simulink library "acc"  (R2021b)
settings: Solver=VariableStepAuto  StartTime=0.0  StopTime=10.0  RelTol=1e-3
undefined symbols (not defined in the file or in its folder): AACC_EHPSSpdCtrlMode_X_enum, AACC_EHPSSpdCtrlMode_Y_rad, ENUM__SASCALED_CALED, ENUM_BRAKEPEDAL_RELEASED, ENUM_CACENABLESTS_RUN, ENUM_DCDCENABLESTS_RUN, ENUM_EHPSCTRLMODE_FULLPWR, ENUM_EHPSCTRLMODE_NORMAL, ENUM_EHPSCTRLMODE_STEP1, ENUM_EHPSCTRLMODE_ZERO, ENUM_EHPSENABLESTS_INITIAL, ENUM_EHPSENABLESTS_READY, ENUM_EHPSENABLESTS_RUN, ENUM_PMMMODE_DRIVE, ENUM_PMMMODE_POWERUP, ENUM_TARGETGEAR_NEUTRAL, FALSE, KACC_AirPressInvalid_kpa, KACC_CACEnableFailTime_s, KACC_CACOverrunRcvTime_s, KACC_CACOverrunTime_min, KACC_CACOverTempDelayTime_s, KACC_CACOverTempRcv_s, KACC_CACPresLow_kPa, KACC_CACPressureSWRev_flg, KACC_CACPresWarn_kPa, KACC_CACPresWarn_ovrdflg_flg, KACC_CACPresWarn_ovrdval_flg, KACC_CACStopTime_s, KACC_CACTemp_C, KACC_CACTempRev_C, KACC_CACTempStop_C, KACC_CACTempWarn_C, KACC_CACValid_flg, KACC_CP2VAutoTracH_enum, KACC_CP2VDamStiffReqFA_pct, KACC_CP2VDamStiffReqLA_pct, KACC_CP2VDamStiffReqRA_pct, KACC_CP2VKneeCtrlMReq_enum, KACC_CP2VKneeReqFA_enum, KACC_CP2VKneeReqRA_enum, KACC_CP2VKneeReqRSide_enum, KACC_CP2VLA1PosCmd_enum, KACC_CP2VLA2PosCmd_enum, KACC_CP2VLvCtrlModeReq_enum, KACC_CP2VNLvReqFA_enum, KACC_CP2VNLvReqRA_enum, KACC_DCDCErrLvHoldtime_s, KACC_DTCACCReset_flg, KACC_DTCCACOverrun_cnt, KACC_EACErrLvHoldtime_s, KACC_ECASKneeSideSW_flg, KACC_EcasSw1Down_flg, KACC_EcasSw1Up_flg, KACC_EcasSw2M2_flg, KACC_EcasSw2Stop_flg, KACC_EcasSw3Knee_flg, KACC_EcasSw3M1_flg, KACC_EcasSwDebounceTime_s, KACC_ECASSwitch_flg ... (+30)
libraries: hcu_lib x20, simulink x3
(part 3 of 3)

== system acc/ACC/OutpConvert/EHPS Enable TimeOut Judgment ==
  BSCP_In_outputs : Inport
  BMain_outputs : Inport  Port=2
  Bus Selector : BusSelector  OutputSignals=VPMM_EHPSIniFinish_flg,VINP_EHPSEnSta_enum,task_time_s
  Bus Selector1 : BusSelector  OutputSignals=VACC_InitEHPSEnDem_flg
  Constant19 : Constant  Value=ENUM_EHPSENABLESTS_INITIAL
  Constant20 : Constant  Value=KACC_EHPSDisableFailTime_s
  Constant21 : Constant  Value=ENUM_EHPSENABLESTS_READY
  DelayEnable1 : Subsystem  mask(DelayEnable){}
      mask help: Delay enable funcion.
  Logical Operator1 : Logic  Inputs=3  AllPortsSameDT=off  OutDataTypeStr=boolean
  Logical Operator3 : Logic  Operator=OR  AllPortsSameDT=off  OutDataTypeStr=boolean
  NOT1 : Logic  Operator=NOT  AllPortsSameDT=off  OutDataTypeStr=boolean
  Relational Operator7 : RelationalOperator  Operator=~=  OutDataTypeStr=boolean  RndMeth=Simplest
  Relational Operator8 : RelationalOperator  Operator=~=  OutDataTypeStr=boolean  RndMeth=Simplest
  Unit Delay3 : UnitDelay  InitialCondition=boolean(0)  SampleTime=-1  HasFrameUpgradeWarning=on
      settings: AttributesFormatString=%<InitialCondition>
  VACC_EHPSDisEnTimeout_flg : Outport
  wires:
  [task_time_s] -> DelayEnable1/3(Ts)
  [VINP_EHPSEnSta_enum] -> Relational Operator8/1
  DelayEnable1/1(set) -> Unit Delay3/1
  Relational Operator7/1 -> Logical Operator3/1
  Constant20/1 -> DelayEnable1/2(T_delay)
  Logical Operator3/1 -> Logical Operator1/3
  Constant21/1 -> Relational Operator8/2
  [VINP_EHPSEnSta_enum] -> Relational Operator7/1
  NOT1/1 -> Logical Operator1/2
  Constant19/1 -> Relational Operator7/2
  [VACC_InitEHPSEnDem_flg] -> NOT1/1
  [VPMM_EHPSIniFinish_flg] -> Logical Operator1/1
  Relational Operator8/1 -> Logical Operator3/2
  Logical Operator1/1 -> DelayEnable1/1(trigger)
  Bus Selector/1 -> [VPMM_EHPSIniFinish_flg]  "<VPMM_EHPSIniFinish_flg>"
  Bus Selector/2 -> [VINP_EHPSEnSta_enum]  "<VINP_EHPSEnSta_enum>"
  BSCP_In_outputs/1 -> Bus Selector/1
  BMain_outputs/1 -> Bus Selector1/1
  Bus Selector1/1 -> [VACC_InitEHPSEnDem_flg]  "<VACC_InitEHPSEnDem_flg>"
  Bus Selector/3 -> [task_time_s]  "<task_time_s>"
  Unit Delay3/1 -> [VACC_EHPSDisEnTimeout_flg]  "VACC_EHPSDisEnTimeout_flg"
  [VACC_EHPSDisEnTimeout_flg] -> VACC_EHPSDisEnTimeout_flg/1

== system acc/ACC/OutpConvert/PCU Demand SCP ==
  BMain_outputs : Inport
  Bus Selector1 : BusSelector  OutputSignals=VACC_EHPSEnableDem_flg,VACC_CACEnableDem_flg,VACC_DCDCEnableDem_flg
  Constant10 : Constant  Value=hex2dec('AA')  OutDataTypeStr=uint8
  Constant11 : Constant  Value=ZERO_FLOAT
  Constant12 : Constant  Value=ZERO_FLOAT
  Constant6 : Constant  Value=hex2dec('55')  OutDataTypeStr=uint8
  Constant7 : Constant  Value=hex2dec('AA')  OutDataTypeStr=uint8
  Constant8 : Constant  Value=hex2dec('55')  OutDataTypeStr=uint8
  Constant9 : Constant  Value=hex2dec('AA')  OutDataTypeStr=uint8
  Constant90 : Constant  Value=hex2dec('55')  OutDataTypeStr=uint8
  Data Type Conversion63 : DataTypeConversion  OutDataTypeStr=single
  Data Type Conversion64 : DataTypeConversion  OutDataTypeStr=single
  Switch : Switch  Criteria=u2 > Threshold
  Switch1 : Switch  Criteria=u2 > Threshold
  Switch2 : Switch  Criteria=u2 > Threshold
  Terminator : Terminator
  VACC_EHPSEnDemand_enum : Outport
  VACC_EACEnDemand_enum : Outport  Port=2
  VACC_DCDCEnDemamd_enum : Outport  Port=3
  VACC_EACSpdDemand_rpm : Outport  Port=4
  wires:
  Constant10/1 -> Switch2/3
  Constant9/1 -> Switch/3
  Constant11/1 -> Data Type Conversion64/1
  Constant6/1 -> Switch1/1
  Constant7/1 -> Switch1/3
  Constant12/1 -> Data Type Conversion63/1
  Data Type Conversion64/1 -> Terminator/1
  Constant90/1 -> Switch2/1
  Constant8/1 -> Switch/1
  BMain_outputs/1 -> Bus Selector1/1
  Bus Selector1/1 -> [VACC_EHPSEnableDem_flg]  "<VACC_EHPSEnableDem_flg>"
  Bus Selector1/2 -> [VACC_CACEnableDem_flg]  "<VACC_CACEnableDem_flg>"
  Bus Selector1/3 -> [VACC_DCDCEnableDem_flg]  "<VACC_DCDCEnableDem_flg>"
  [VACC_EHPSEnableDem_flg] -> Switch/2
  [VACC_DCDCEnableDem_flg] -> Switch2/2
  [VACC_CACEnableDem_flg] -> Switch1/2
  Switch/1 -> [VACC_EHPSEnDemand_enum]  "VACC_EHPSEnDemand_enum"
  Switch1/1 -> [VACC_EACEnDemand_enum]  "VACC_EACEnDemand_enum"
  Switch2/1 -> [VACC_DCDCEnDemamd_enum]  "VACC_DCDCEnDemamd_enum"
  Data Type Conversion63/1 -> [VACC_EACSpdDemand_rpm]  "VACC_EACSpdDemand_rpm"
  [VACC_EHPSEnDemand_enum] -> VACC_EHPSEnDemand_enum/1
  [VACC_EACEnDemand_enum] -> VACC_EACEnDemand_enum/1
  [VACC_DCDCEnDemamd_enum] -> VACC_DCDCEnDemamd_enum/1
  [VACC_EACSpdDemand_rpm] -> VACC_EACSpdDemand_rpm/1

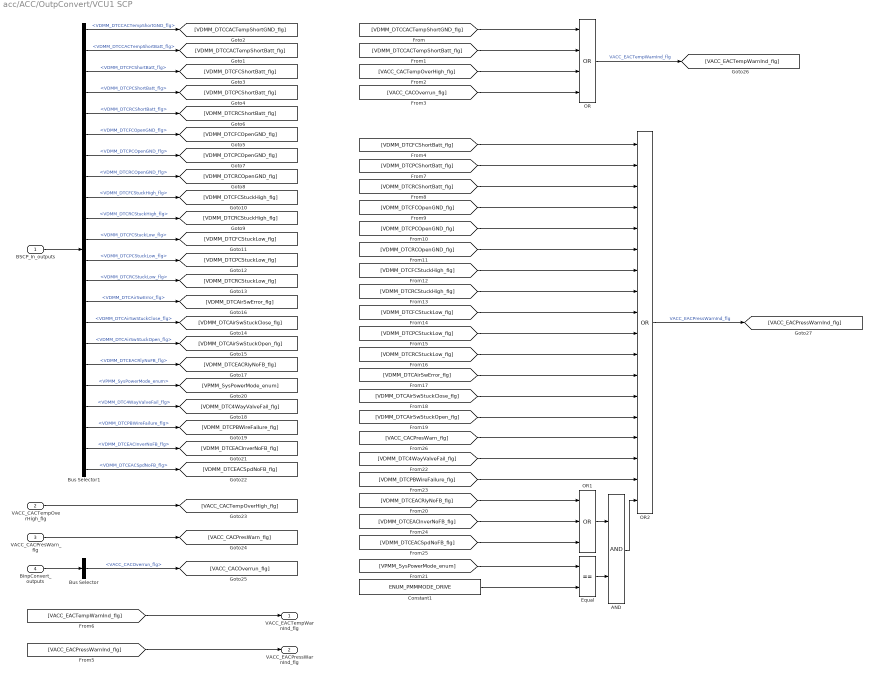
== system acc/ACC/OutpConvert/VCU1 SCP ==
  BSCP_In_outputs : Inport
  VACC_CACTempOverHigh_flg : Inport  Port=2
  VACC_CACPresWarn_flg : Inport  Port=3
  BInpConvert_outputs : Inport  Port=4
  AND : Logic  AllPortsSameDT=off  OutDataTypeStr=boolean
  Bus Selector : BusSelector  OutputSignals=VACC_CACOverrun_flg
  Bus Selector1 : BusSelector  OutputSignals=VDMM_DTCCACTempShortGND_flg,VDMM_DTCCACTempShortBatt_flg,VDMM_DTCFCShortBatt_flg,VDMM_DTCPCShortBatt_flg,VDMM_DTCRCShortBatt_flg,VDMM_DTCFCOpenGND_flg,VDMM_DTCPCOpenGND_flg,VDMM_DTCRCOpenGND_flg,VDMM_DTCFCStuckHigh_flg,VDMM_DTCRCStuckHigh_flg,VDMM_DTCFCStuckLow_flg,VDMM_DTCPCStuckLow_flg,VDMM_DTCRCStuckLow_flg,VDMM_DTCAirSwError_flg,VDMM_DTCAirSwStuckClose_flg,VDMM_DTCAirSwStuckOpen_flg,VDMM_DTCEACRlyNoFB_flg,VPMM_SysPowerMode_enum,VDMM_DTC4WayValveFail_flg,VDMM_DTCPBWireFailure_flg,VDMM_DTCEACInverNoFB_flg,VDMM_DTCEACSpdNoFB_flg
  Constant1 : Constant  Value=ENUM_PMMMODE_DRIVE
  Equal : RelationalOperator  Operator===  OutDataTypeStr=boolean  RndMeth=Simplest
  OR : Logic  Operator=OR  Inputs=4  AllPortsSameDT=off  OutDataTypeStr=boolean
  OR1 : Logic  Operator=OR  Inputs=3  AllPortsSameDT=off  OutDataTypeStr=boolean
  OR2 : Logic  Operator=OR  Inputs=18  AllPortsSameDT=off  OutDataTypeStr=boolean
  VACC_EACTempWarnInd_flg : Outport
  VACC_EACPressWarnInd_flg : Outport  Port=2
  wires:
  [VACC_EACPressWarnInd_flg] -> VACC_EACPressWarnInd_flg/1
  [VACC_EACTempWarnInd_flg] -> VACC_EACTempWarnInd_flg/1
  BSCP_In_outputs/1 -> Bus Selector1/1
  Bus Selector1/4 -> [VDMM_DTCPCShortBatt_flg]  "<VDMM_DTCPCShortBatt_flg>"
  Bus Selector1/3 -> [VDMM_DTCFCShortBatt_flg]  "<VDMM_DTCFCShortBatt_flg>"
  Bus Selector1/2 -> [VDMM_DTCCACTempShortBatt_flg]  "<VDMM_DTCCACTempShortBatt_flg>"
  Bus Selector1/1 -> [VDMM_DTCCACTempShortGND_flg]  "<VDMM_DTCCACTempShortGND_flg>"
  Bus Selector1/5 -> [VDMM_DTCRCShortBatt_flg]  "<VDMM_DTCRCShortBatt_flg>"
  Bus Selector1/6 -> [VDMM_DTCFCOpenGND_flg]  "<VDMM_DTCFCOpenGND_flg>"
  Bus Selector1/7 -> [VDMM_DTCPCOpenGND_flg]  "<VDMM_DTCPCOpenGND_flg>"
  Bus Selector1/8 -> [VDMM_DTCRCOpenGND_flg]  "<VDMM_DTCRCOpenGND_flg>"
  Bus Selector1/9 -> [VDMM_DTCFCStuckHigh_flg]  "<VDMM_DTCFCStuckHigh_flg>"
  Bus Selector1/10 -> [VDMM_DTCRCStuckHigh_flg]  "<VDMM_DTCRCStuckHigh_flg>"
  Bus Selector1/11 -> [VDMM_DTCFCStuckLow_flg]  "<VDMM_DTCFCStuckLow_flg>"
  Bus Selector1/12 -> [VDMM_DTCPCStuckLow_flg]  "<VDMM_DTCPCStuckLow_flg>"
  Bus Selector1/13 -> [VDMM_DTCRCStuckLow_flg]  "<VDMM_DTCRCStuckLow_flg>"
  Bus Selector1/14 -> [VDMM_DTCAirSwError_flg]  "<VDMM_DTCAirSwError_flg>"
  Bus Selector1/15 -> [VDMM_DTCAirSwStuckClose_flg]  "<VDMM_DTCAirSwStuckClose_flg>"
  Bus Selector1/16 -> [VDMM_DTCAirSwStuckOpen_flg]  "<VDMM_DTCAirSwStuckOpen_flg>"
  Bus Selector1/17 -> [VDMM_DTCEACRlyNoFB_flg]  "<VDMM_DTCEACRlyNoFB_flg>"
  Bus Selector1/18 -> [VPMM_SysPowerMode_enum]  "<VPMM_SysPowerMode_enum>"
  Bus Selector1/19 -> [VDMM_DTC4WayValveFail_flg]  "<VDMM_DTC4WayValveFail_flg>"
  Bus Selector1/20 -> [VDMM_DTCPBWireFailure_flg]  "<VDMM_DTCPBWireFailure_flg>"
  Bus Selector1/21 -> [VDMM_DTCEACInverNoFB_flg]  "<VDMM_DTCEACInverNoFB_flg>"
  Bus Selector1/22 -> [VDMM_DTCEACSpdNoFB_flg]  "<VDMM_DTCEACSpdNoFB_flg>"
  BInpConvert_outputs/1 -> Bus Selector/1
  Bus Selector/1 -> [VACC_CACOverrun_flg]  "<VACC_CACOverrun_flg>"
  VACC_CACPresWarn_flg/1 -> [VACC_CACPresWarn_flg]
  VACC_CACTempOverHigh_flg/1 -> [VACC_CACTempOverHigh_flg]
  [VDMM_DTCCACTempShortGND_flg] -> OR/1
  [VDMM_DTCCACTempShortBatt_flg] -> OR/2
  [VACC_CACTempOverHigh_flg] -> OR/3
  [VACC_CACOverrun_flg] -> OR/4
  OR/1 -> [VACC_EACTempWarnInd_flg]  "VACC_EACTempWarnInd_flg"
  Constant1/1 -> Equal/2
  [VPMM_SysPowerMode_enum] -> Equal/1
  [VDMM_DTCEACRlyNoFB_flg] -> OR1/1
  [VDMM_DTCEACInverNoFB_flg] -> OR1/2
  [VDMM_DTCEACSpdNoFB_flg] -> OR1/3
  OR1/1 -> AND/1
  Equal/1 -> AND/2
  [VDMM_DTCFCShortBatt_flg] -> OR2/1
  [VDMM_DTCPCShortBatt_flg] -> OR2/2
  [VDMM_DTCRCShortBatt_flg] -> OR2/3
  [VDMM_DTCFCOpenGND_flg] -> OR2/4
  [VDMM_DTCPCOpenGND_flg] -> OR2/5
  [VDMM_DTCRCOpenGND_flg] -> OR2/6
  [VDMM_DTCFCStuckHigh_flg] -> OR2/7
  [VDMM_DTCRCStuckHigh_flg] -> OR2/8
  [VDMM_DTCFCStuckLow_flg] -> OR2/9
  [VDMM_DTCPCStuckLow_flg] -> OR2/10
  [VDMM_DTCRCStuckLow_flg] -> OR2/11
  [VDMM_DTCAirSwError_flg] -> OR2/12
  [VDMM_DTCAirSwStuckClose_flg] -> OR2/13
  [VDMM_DTCAirSwStuckOpen_flg] -> OR2/14
  [VACC_CACPresWarn_flg] -> OR2/15
  [VDMM_DTC4WayValveFail_flg] -> OR2/16
  [VDMM_DTCPBWireFailure_flg] -> OR2/17
  AND/1 -> OR2/18
  OR2/1 -> [VACC_EACPressWarnInd_flg]  "VACC_EACPressWarnInd_flg"

== system acc/ACC/OutpConvert/VCU5 SCP ==
  BSCP_In_outputs : Inport
  Bus Selector1 : BusSelector  OutputSignals=VINP_CACTemp_C,VINP_FDCCHASSISVCUEACPressSta_flg,VDMM_DTCCACTempShortGND_flg,VDMM_DTCCACTempShortBatt_flg
  Constant1 : Constant  Value=KACC_CACPressureSWRev_flg
  Constant21 : Constant  Value=KACC_VCUEACpumpTempInvalid_C
  NOT : Logic  Operator=NOT  AllPortsSameDT=off  OutDataTypeStr=boolean
  OR : Logic  Operator=OR  AllPortsSameDT=off  OutDataTypeStr=boolean
  Switch : Switch  Criteria=u2 ~= 0
      settings: AttributesFormatString=%<Criteria>
  Switch1 : Switch  Criteria=u2 ~= 0
      settings: AttributesFormatString=%<Criteria>
  VACC_VCUEACpumpTemp_C : Outport
  VACC_VCUEACPressureSW_flg : Outport  Port=2
  wires:
  BSCP_In_outputs/1 -> Bus Selector1/1
  Bus Selector1/1 -> [VINP_CACTemp_C]  "<VINP_CACTemp_C>"
  Bus Selector1/2 -> [VINP_FDCCHASSISVCUEACPressSta_flg]  "<VINP_FDCCHASSISVCUEACPressSta_flg>"
  Bus Selector1/3 -> [VDMM_DTCCACTempShortGND_flg]  "<VDMM_DTCCACTempShortGND_flg>"
  Bus Selector1/4 -> [VDMM_DTCCACTempShortBatt_flg]  "<VDMM_DTCCACTempShortBatt_flg>"
  OR/1 -> Switch/2
  [VDMM_DTCCACTempShortGND_flg] -> OR/1
  [VDMM_DTCCACTempShortBatt_flg] -> OR/2
  Constant21/1 -> Switch/1
  [VINP_CACTemp_C] -> Switch/3
  Switch/1 -> [VACC_VCUEACpumpTemp_C]  "VACC_VCUEACpumpTemp_C"
  Constant1/1 -> Switch1/2
  [VINP_FDCCHASSISVCUEACPressSta_flg] -> NOT/1
  NOT/1 -> Switch1/3
  [VINP_FDCCHASSISVCUEACPressSta_flg] -> Switch1/1
  Switch1/1 -> [VACC_VCUEACPressureSW_flg]  "VACC_VCUEACPressureSW_flg"
  [VACC_VCUEACpumpTemp_C] -> VACC_VCUEACpumpTemp_C/1
  [VACC_VCUEACPressureSW_flg] -> VACC_VCUEACPressureSW_flg/1

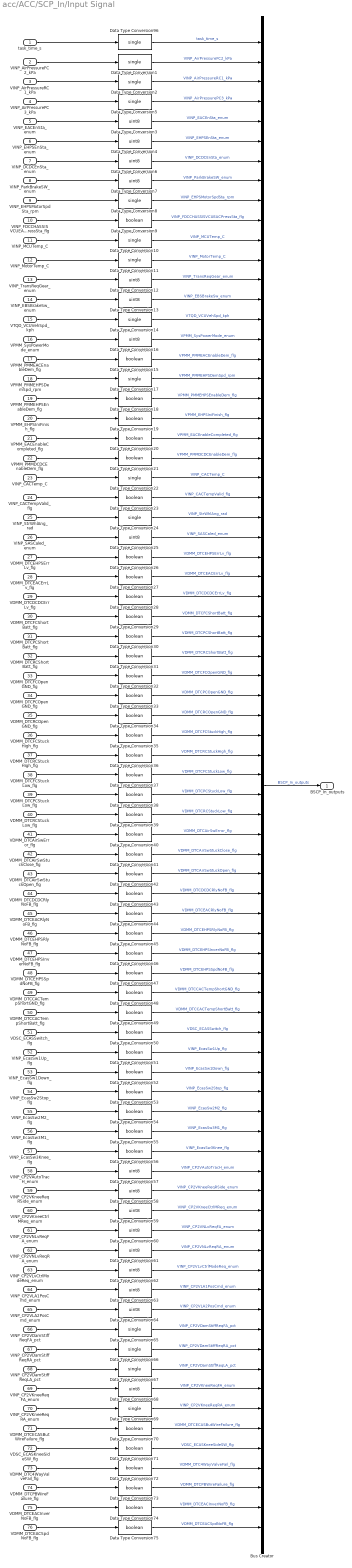
== system acc/ACC/SCP_In/Input Signal ==
  task_time_s : Inport
  VINP_AirPressureFC2_kPa : Inport  Port=2
  VINP_AirPressureRC1_kPa : Inport  Port=3
  VINP_AirPressurePC3_kPa : Inport  Port=4
  VINP_EACEnSta_enum : Inport  Port=5
  VINP_EHPSEnSta_enum : Inport  Port=6
  VINP_DCDCEnSta_enum : Inport  Port=7
  VINP_ParkBrakeSW_enum : Inport  Port=8
  VINP_EHPSMotorSpdSta_rpm : Inport  Port=9
  VINP_FDCCHASSISVCUEACPressSta_flg : Inport  Port=10
  VINP_MCUTemp_C : Inport  Port=11
  VINP_MotorTemp_C : Inport  Port=12
  VINP_TransReqGear_enum : Inport  Port=13
  VINP_EBSBrakeSw_enum : Inport  Port=14
  VTQD_VCUVehSpd_kph : Inport  Port=15
  VPMM_SysPowerMode_enum : Inport  Port=16
  VPMM_PMMEACEnableDem_flg : Inport  Port=17
  VPMM_PMMEHPSDemSpd_rpm : Inport  Port=18
  VPMM_PMMEHPSEnableDem_flg : Inport  Port=19
  VPMM_EHPSIniFinish_flg : Inport  Port=20
  VPMM_EACEnableCompleted_flg : Inport  Port=21
  VPMM_PMMDCDCEnableDem_flg : Inport  Port=22
  VINP_CACTemp_C : Inport  Port=23
  VINP_CACTempValid_flg : Inport  Port=24
  VINP_StrWhlAng_rad : Inport  Port=25
  VINP_SASCaled_enum : Inport  Port=26
  VDMM_DTCEHPSErrLv_flg : Inport  Port=27
  VDMM_DTCEACErrLv_flg : Inport  Port=28
  VDMM_DTCDCDCErrLv_flg : Inport  Port=29
  VDMM_DTCFCShortBatt_flg : Inport  Port=30
  VDMM_DTCPCShortBatt_flg : Inport  Port=31
  VDMM_DTCRCShortBatt_flg : Inport  Port=32
  VDMM_DTCFCOpenGND_flg : Inport  Port=33
  VDMM_DTCPCOpenGND_flg : Inport  Port=34
  VDMM_DTCRCOpenGND_flg : Inport  Port=35
  VDMM_DTCFCStuckHigh_flg : Inport  Port=36
  VDMM_DTCRCStuckHigh_flg : Inport  Port=37
  VDMM_DTCFCStuckLow_flg : Inport  Port=38
  VDMM_DTCPCStuckLow_flg : Inport  Port=39
  VDMM_DTCRCStuckLow_flg : Inport  Port=40
  VDMM_DTCAirSwError_flg : Inport  Port=41
  VDMM_DTCAirSwStuckClose_flg : Inport  Port=42
  VDMM_DTCAirSwStuckOpen_flg : Inport  Port=43
  VDMM_DTCDCDCRlyNoFB_flg : Inport  Port=44
  VDMM_DTCEACRlyNoFB_flg : Inport  Port=45
  VDMM_DTCEHPSRlyNoFB_flg : Inport  Port=46
  VDMM_DTCEHPSInverNoFB_flg : Inport  Port=47
  VDMM_DTCEHPSSpdNoFB_flg : Inport  Port=48
  VDMM_DTCCACTempShortGND_flg : Inport  Port=49
  VDMM_DTCCACTempShortBatt_flg : Inport  Port=50
  VDSC_ECASSwitch_flg : Inport  Port=51
  VINP_EcasSw1Up_flg : Inport  Port=52
  VINP_EcasSw1Down_flg : Inport  Port=53
  VINP_EcasSw2Stop_flg : Inport  Port=54
  VINP_EcasSw2M2_flg : Inport  Port=55
  VINP_EcasSw3M1_flg : Inport  Port=56
  VINP_EcasSw3Knee_flg : Inport  Port=57
  VINP_CP2VAutoTracH_enum : Inport  Port=58
  VINP_CP2VKneeReqRSide_enum : Inport  Port=59
  VINP_CP2VKneeCtrlMReq_enum : Inport  Port=60
  VINP_CP2VNLvReqFA_enum : Inport  Port=61
  VINP_CP2VNLvReqRA_enum : Inport  Port=62
  VINP_CP2VLvCtrlModeReq_enum : Inport  Port=63
  VINP_CP2VLA1PosCmd_enum : Inport  Port=64
  VINP_CP2VLA2PosCmd_enum : Inport  Port=65
  VINP_CP2VDamStiffReqFA_pct : Inport  Port=66
  VINP_CP2VDamStiffReqRA_pct : Inport  Port=67
  VINP_CP2VDamStiffReqLA_pct : Inport  Port=68
  VINP_CP2VKneeReqFA_enum : Inport  Port=69
  VINP_CP2VKneeReqRA_enum : Inport  Port=70
  VDMM_DTCECASButWireFailure_flg : Inport  Port=71
  VDSC_ECASKneeSideSW_flg : Inport  Port=72
  VDMM_DTC4WayValveFail_flg : Inport  Port=73
  VDMM_DTCPBWireFailure_flg : Inport  Port=74
  VDMM_DTCEACInverNoFB_flg : Inport  Port=75
  VDMM_DTCEACSpdNoFB_flg : Inport  Port=76
  Bus Creator : BusCreator  Inputs=76
  Data Type Conversion{1..2,5,8,10..11,14,17,22,24,65..67,69,96} (15 alike) : DataTypeConversion  OutDataTypeStr=single
  Data Type Conversion{3..4,6..7,12..13,16,25,57..64,68} (17 alike) : DataTypeConversion  OutDataTypeStr=uint8
  Data Type Conversion{9,15,18..21,23,26..56,70..75} (44 alike) : DataTypeConversion  OutDataTypeStr=boolean
  BSCP_In_outputs : Outport
  wires:
  Data Type Conversion5/1 -> Bus Creator/4  "VINP_AirPressurePC3_kPa"
  Data Type Conversion2/1 -> Bus Creator/3  "VINP_AirPressureRC1_kPa"
  Data Type Conversion1/1 -> Bus Creator/2  "VINP_AirPressureFC2_kPa"
  VDMM_DTCPCStuckLow_flg/1 -> Data Type Conversion38/1
  Data Type Conversion41/1 -> Bus Creator/42  "VDMM_DTCAirSwStuckClose_flg"
  Data Type Conversion7/1 -> Bus Creator/8  "VINP_ParkBrakeSW_enum"
  Data Type Conversion29/1 -> Bus Creator/30  "VDMM_DTCFCShortBatt_flg"
  VINP_EHPSEnSta_enum/1 -> Data Type Conversion4/1
  Data Type Conversion37/1 -> Bus Creator/38  "VDMM_DTCFCStuckLow_flg"
  Data Type Conversion3/1 -> Bus Creator/5  "VINP_EACEnSta_enum"
  Data Type Conversion42/1 -> Bus Creator/43  "VDMM_DTCAirSwStuckOpen_flg"
  VINP_FDCCHASSISVCUEACPressSta_flg/1 -> Data Type Conversion9/1
  Data Type Conversion24/1 -> Bus Creator/25  "VINP_StrWhlAng_rad"
  Data Type Conversion8/1 -> Bus Creator/9  "VINP_EHPSMotorSpdSta_rpm"
  Data Type Conversion26/1 -> Bus Creator/27  "VDMM_DTCEHPSErrLv_flg"
  task_time_s/1 -> Data Type Conversion96/1
  VDMM_DTCAirSwError_flg/1 -> Data Type Conversion40/1
  Data Type Conversion34/1 -> Bus Creator/35  "VDMM_DTCRCOpenGND_flg"
  Data Type Conversion4/1 -> Bus Creator/6  "VINP_EHPSEnSta_enum"
  Data Type Conversion12/1 -> Bus Creator/13  "VINP_TransReqGear_enum"
  Data Type Conversion11/1 -> Bus Creator/12  "VINP_MotorTemp_C"
  Data Type Conversion6/1 -> Bus Creator/7  "VINP_DCDCEnSta_enum"
  VPMM_SysPowerMode_enum/1 -> Data Type Conversion16/1
  Data Type Conversion33/1 -> Bus Creator/34  "VDMM_DTCPCOpenGND_flg"
  Data Type Conversion28/1 -> Bus Creator/29  "VDMM_DTCDCDCErrLv_flg"
  VINP_AirPressureRC1_kPa/1 -> Data Type Conversion2/1
  Data Type Conversion9/1 -> Bus Creator/10  "VINP_FDCCHASSISVCUEACPressSta_flg"
  VINP_DCDCEnSta_enum/1 -> Data Type Conversion6/1
  Data Type Conversion10/1 -> Bus Creator/11  "VINP_MCUTemp_C"
  Data Type Conversion45/1 -> Bus Creator/46  "VDMM_DTCEHPSRlyNoFB_flg"
  VINP_SASCaled_enum/1 -> Data Type Conversion25/1
  Data Type Conversion16/1 -> Bus Creator/16  "VPMM_SysPowerMode_enum"
  VDMM_DTCPCOpenGND_flg/1 -> Data Type Conversion33/1
  Data Type Conversion14/1 -> Bus Creator/15  "VTQD_VCUVehSpd_kph"
  Data Type Conversion36/1 -> Bus Creator/37  "VDMM_DTCRCStuckHigh_flg"
  VINP_AirPressurePC3_kPa/1 -> Data Type Conversion5/1
  Data Type Conversion15/1 -> Bus Creator/17  "VPMM_PMMEACEnableDem_flg"
  Data Type Conversion17/1 -> Bus Creator/18  "VPMM_PMMEHPSDemSpd_rpm"
  VDMM_DTCEHPSSpdNoFB_flg/1 -> Data Type Conversion47/1
  Data Type Conversion13/1 -> Bus Creator/14  "VINP_EBSBrakeSw_enum"
  Bus Creator/1 -> BSCP_In_outputs/1  "BSCP_In_outputs"
  VTQD_VCUVehSpd_kph/1 -> Data Type Conversion14/1
  Data Type Conversion21/1 -> Bus Creator/22  "VPMM_PMMDCDCEnableDem_flg"
  Data Type Conversion19/1 -> Bus Creator/20  "VPMM_EHPSIniFinish_flg"
  Data Type Conversion18/1 -> Bus Creator/19  "VPMM_PMMEHPSEnableDem_flg"
  Data Type Conversion39/1 -> Bus Creator/40  "VDMM_DTCRCStuckLow_flg"
  Data Type Conversion43/1 -> Bus Creator/44  "VDMM_DTCDCDCRlyNoFB_flg"
  Data Type Conversion22/1 -> Bus Creator/23  "VINP_CACTemp_C"
  VDMM_DTCDCDCErrLv_flg/1 -> Data Type Conversion28/1
  Data Type Conversion20/1 -> Bus Creator/21  "VPMM_EACEnableCompleted_flg"
  VINP_ParkBrakeSW_enum/1 -> Data Type Conversion7/1
  Data Type Conversion27/1 -> Bus Creator/28  "VDMM_DTCEACErrLv_flg"
  VDMM_DTCRCStuckHigh_flg/1 -> Data Type Conversion36/1
  Data Type Conversion30/1 -> Bus Creator/31  "VDMM_DTCPCShortBatt_flg"
  Data Type Conversion25/1 -> Bus Creator/26  "VINP_SASCaled_enum"
  Data Type Conversion23/1 -> Bus Creator/24  "VINP_CACTempValid_flg"
  Data Type Conversion31/1 -> Bus Creator/32  "VDMM_DTCRCShortBatt_flg"
  Data Type Conversion32/1 -> Bus Creator/33  "VDMM_DTCFCOpenGND_flg"
  Data Type Conversion35/1 -> Bus Creator/36  "VDMM_DTCFCStuckHigh_flg"
  Data Type Conversion38/1 -> Bus Creator/39  "VDMM_DTCPCStuckLow_flg"
  Data Type Conversion40/1 -> Bus Creator/41  "VDMM_DTCAirSwError_flg"
  VDMM_DTCRCShortBatt_flg/1 -> Data Type Conversion31/1
  Data Type Conversion47/1 -> Bus Creator/48  "VDMM_DTCEHPSSpdNoFB_flg"
  VINP_CACTemp_C/1 -> Data Type Conversion22/1
  Data Type Conversion46/1 -> Bus Creator/47  "VDMM_DTCEHPSInverNoFB_flg"
  Data Type Conversion44/1 -> Bus Creator/45  "VDMM_DTCEACRlyNoFB_flg"
  Data Type Conversion96/1 -> Bus Creator/1  "task_time_s"
  VINP_EBSBrakeSw_enum/1 -> Data Type Conversion13/1
  VINP_EHPSMotorSpdSta_rpm/1 -> Data Type Conversion8/1
  VDMM_DTCAirSwStuckOpen_flg/1 -> Data Type Conversion42/1
  VDMM_DTCFCShortBatt_flg/1 -> Data Type Conversion29/1
  VPMM_EACEnableCompleted_flg/1 -> Data Type Conversion20/1
  VINP_EACEnSta_enum/1 -> Data Type Conversion3/1
  VDMM_DTCEACRlyNoFB_flg/1 -> Data Type Conversion44/1
  VDMM_DTCDCDCRlyNoFB_flg/1 -> Data Type Conversion43/1
  VDMM_DTCEHPSRlyNoFB_flg/1 -> Data Type Conversion45/1
  VDMM_DTCRCStuckLow_flg/1 -> Data Type Conversion39/1
  VINP_CACTempValid_flg/1 -> Data Type Conversion23/1
  VPMM_EHPSIniFinish_flg/1 -> Data Type Conversion19/1
  VPMM_PMMEHPSEnableDem_flg/1 -> Data Type Conversion18/1
  VDMM_DTCEHPSInverNoFB_flg/1 -> Data Type Conversion46/1
  VINP_TransReqGear_enum/1 -> Data Type Conversion12/1
  VDMM_DTCPCShortBatt_flg/1 -> Data Type Conversion30/1
  VINP_AirPressureFC2_kPa/1 -> Data Type Conversion1/1
  VDMM_DTCRCOpenGND_flg/1 -> Data Type Conversion34/1
  VDMM_DTCFCStuckHigh_flg/1 -> Data Type Conversion35/1
  VDMM_DTCFCOpenGND_flg/1 -> Data Type Conversion32/1
  VINP_StrWhlAng_rad/1 -> Data Type Conversion24/1
  VDMM_DTCEHPSErrLv_flg/1 -> Data Type Conversion26/1
  VPMM_PMMDCDCEnableDem_flg/1 -> Data Type Conversion21/1
  VPMM_PMMEHPSDemSpd_rpm/1 -> Data Type Conversion17/1
  VDMM_DTCEACErrLv_flg/1 -> Data Type Conversion27/1
  VDMM_DTCAirSwStuckClose_flg/1 -> Data Type Conversion41/1
  VDMM_DTCFCStuckLow_flg/1 -> Data Type Conversion37/1
  VPMM_PMMEACEnableDem_flg/1 -> Data Type Conversion15/1
  VINP_MCUTemp_C/1 -> Data Type Conversion10/1
  VINP_MotorTemp_C/1 -> Data Type Conversion11/1
  VDMM_DTCCACTempShortGND_flg/1 -> Data Type Conversion48/1
  VDMM_DTCCACTempShortBatt_flg/1 -> Data Type Conversion49/1
  Data Type Conversion48/1 -> Bus Creator/49  "VDMM_DTCCACTempShortGND_flg"
  Data Type Conversion49/1 -> Bus Creator/50  "VDMM_DTCCACTempShortBatt_flg"
  VDSC_ECASSwitch_flg/1 -> Data Type Conversion50/1
  Data Type Conversion50/1 -> Bus Creator/51  "VDSC_ECASSwitch_flg"
  VINP_EcasSw1Up_flg/1 -> Data Type Conversion51/1
  VINP_EcasSw1Down_flg/1 -> Data Type Conversion52/1
  VINP_EcasSw2M2_flg/1 -> Data Type Conversion54/1
  VINP_EcasSw2Stop_flg/1 -> Data Type Conversion53/1
  VINP_EcasSw3M1_flg/1 -> Data Type Conversion55/1
  VINP_EcasSw3Knee_flg/1 -> Data Type Conversion56/1
  Data Type Conversion51/1 -> Bus Creator/52  "VINP_EcasSw1Up_flg"
  Data Type Conversion52/1 -> Bus Creator/53  "VINP_EcasSw1Down_flg"
  Data Type Conversion53/1 -> Bus Creator/54  "VINP_EcasSw2Stop_flg"
  Data Type Conversion54/1 -> Bus Creator/55  "VINP_EcasSw2M2_flg"
  Data Type Conversion55/1 -> Bus Creator/56  "VINP_EcasSw3M1_flg"
  Data Type Conversion56/1 -> Bus Creator/57  "VINP_EcasSw3Knee_flg"
  VINP_CP2VAutoTracH_enum/1 -> Data Type Conversion57/1
  VINP_CP2VKneeReqRSide_enum/1 -> Data Type Conversion58/1
  VINP_CP2VKneeCtrlMReq_enum/1 -> Data Type Conversion59/1
  VINP_CP2VNLvReqFA_enum/1 -> Data Type Conversion60/1
  VINP_CP2VNLvReqRA_enum/1 -> Data Type Conversion61/1
  VINP_CP2VLvCtrlModeReq_enum/1 -> Data Type Conversion62/1
  VINP_CP2VLA1PosCmd_enum/1 -> Data Type Conversion63/1
  VINP_CP2VLA2PosCmd_enum/1 -> Data Type Conversion64/1
  VINP_CP2VDamStiffReqFA_pct/1 -> Data Type Conversion65/1
  VINP_CP2VDamStiffReqRA_pct/1 -> Data Type Conversion66/1
  VINP_CP2VDamStiffReqLA_pct/1 -> Data Type Conversion67/1
  VINP_CP2VKneeReqFA_enum/1 -> Data Type Conversion68/1
  VINP_CP2VKneeReqRA_enum/1 -> Data Type Conversion69/1
  VDMM_DTCECASButWireFailure_flg/1 -> Data Type Conversion70/1
  Data Type Conversion57/1 -> Bus Creator/58  "VINP_CP2VAutoTracH_enum"
  Data Type Conversion58/1 -> Bus Creator/59  "VINP_CP2VKneeReqRSide_enum"
  Data Type Conversion59/1 -> Bus Creator/60  "VINP_CP2VKneeCtrlMReq_enum"
  Data Type Conversion60/1 -> Bus Creator/61  "VINP_CP2VNLvReqFA_enum"
  Data Type Conversion61/1 -> Bus Creator/62  "VINP_CP2VNLvReqRA_enum"
  Data Type Conversion62/1 -> Bus Creator/63  "VINP_CP2VLvCtrlModeReq_enum"
  Data Type Conversion63/1 -> Bus Creator/64  "VINP_CP2VLA1PosCmd_enum"
  Data Type Conversion64/1 -> Bus Creator/65  "VINP_CP2VLA2PosCmd_enum"
  Data Type Conversion65/1 -> Bus Creator/66  "VINP_CP2VDamStiffReqFA_pct"
  Data Type Conversion66/1 -> Bus Creator/67  "VINP_CP2VDamStiffReqRA_pct"
  Data Type Conversion67/1 -> Bus Creator/68  "VINP_CP2VDamStiffReqLA_pct"
  Data Type Conversion68/1 -> Bus Creator/69  "VINP_CP2VKneeReqFA_enum"
  Data Type Conversion69/1 -> Bus Creator/70  "VINP_CP2VKneeReqRA_enum"
  Data Type Conversion70/1 -> Bus Creator/71  "VDMM_DTCECASButWireFailure_flg"
  VDSC_ECASKneeSideSW_flg/1 -> Data Type Conversion71/1
  Data Type Conversion71/1 -> Bus Creator/72  "VDSC_ECASKneeSideSW_flg"
  VDMM_DTC4WayValveFail_flg/1 -> Data Type Conversion72/1
  VDMM_DTCPBWireFailure_flg/1 -> Data Type Conversion73/1
  VDMM_DTCEACInverNoFB_flg/1 -> Data Type Conversion74/1
  VDMM_DTCEACSpdNoFB_flg/1 -> Data Type Conversion75/1
  Data Type Conversion72/1 -> Bus Creator/73  "VDMM_DTC4WayValveFail_flg"
  Data Type Conversion73/1 -> Bus Creator/74  "VDMM_DTCPBWireFailure_flg"
  Data Type Conversion74/1 -> Bus Creator/75  "VDMM_DTCEACInverNoFB_flg"
  Data Type Conversion75/1 -> Bus Creator/76  "VDMM_DTCEACSpdNoFB_flg"

== system acc/ACC/SCP_In/Invalid Condition ==

== system acc/ACC/OutpConvert/EHPS Enable TimeOut Judgment/DelayEnable1 ==
  trigger : Inport
  T_delay : Inport  Port=2
  Ts : Inport  Port=3
  Constant1 : Constant  Value=ZERO_FLOAT
  Constant2 : Constant  Value=ZERO_FLOAT
  Relational Operator1 : RelationalOperator  Operator=>  OutDataTypeStr=boolean  RndMeth=Nearest
  Subtract1 : Sum
  Switch : Switch  Criteria=u2 ~= 0
      settings: AttributesFormatString=<%<Criteria>>
  Switch1 : Switch  Criteria=u2 ~= 0
      settings: AttributesFormatString=<%<Criteria>>
  Unit Delay : UnitDelay  SampleTime=-1  HasFrameUpgradeWarning=on
      settings: AttributesFormatString=<intial = %<X0>>
  Unit Delay1 : UnitDelay  InitialCondition=FALSE  SampleTime=-1  HasFrameUpgradeWarning=on
      settings: AttributesFormatString=<intial = %<X0>>
  set : Outport
  wires:
  Unit Delay1/1 -> Switch1/2
  Constant2/1 -> Switch1/1
  Ts/1 -> Switch1/3
  Switch1/1 -> Subtract1/2
  Unit Delay/1 -> Subtract1/1
  Relational Operator1/1 -> Unit Delay1/1, set/1
  trigger/1 -> Switch/2
  T_delay/1 -> Relational Operator1/2
  Constant1/1 -> Switch/3
  Switch/1 -> Unit Delay/1, Relational Operator1/1
  Subtract1/1 -> Switch/1

== stateflow chart acc/ACC/Main/EHPS Control/EHPS Control Mode ==
  state Step2
    state ini
      en:
      VACC_EHPSSpdCtrlMode_enum  = ENUM_EHPSCTRLMODE_ZERO;
      VACC_InitEHPSEnDem_flg = FALSE;
    state Normal
      en:
      VACC_EHPSSpdCtrlMode_enum  = ENUM_EHPSCTRLMODE_NORMAL;
      VACC_InitEHPSEnDem_flg = TRUE;
    state BrakePedalPress
      en:
      VACC_EHPSSpdCtrlMode_enum  = ENUM_EHPSCTRLMODE_ZERO;
      VACC_InitEHPSEnDem_flg = TRUE;
    state Still
      en:
      VACC_EHPSSpdCtrlMode_enum  = ENUM_EHPSCTRLMODE_ZERO;
      (default) -> (junction 51) : {
          | cnt = 0;
          | }
      Still -> (junction 51) [order 1]
      (junction 51) -> (junction 57) [order 1] : [VINP_EHPSMotorSpdSta_rpm <= KACC_EHPSSpdDiv_rpm]
      (junction 51) -> (junction 54) [order 2]
      (junction 57) -> (junction 56) : {
          | cnt += task_time_s;
          | }
      (junction 56) -> (junction 54) [order 2]
      (junction 56) -> (junction 58) [order 1] : [cnt >= KACC_EHPSDisWaitTime_s]
      (junction 54) -> (junction 55) : {
          | VACC_InitEHPSEnDem_flg = TRUE;
          | }
      (junction 58) -> (junction 59) : {
          | VACC_InitEHPSEnDem_flg = FALSE;
          | cnt = KACC_EHPSDisWaitTime_s;
          | }
      (junction 59) -> (junction 55)
    state Error
      en:
      VACC_EHPSSpdCtrlMode_enum  = ENUM_EHPSCTRLMODE_FULLPWR;
      VACC_InitEHPSEnDem_flg = TRUE;
    BrakePedalPress -> Normal [order 1] : [!VACC_EHPSDisable_flg]
    ini -> Normal [order 1] : [(VACC_SASCalFinish_flg) && (VPMM_EHPSIniFinish_flg)]
    Still -> BrakePedalPress [order 2] : [(!VACC_EBSBrakeRelease_flg)]
    BrakePedalPress -> Still [order 2] : [VACC_EBSBrakeRelease_flg]
    Normal -> Still [order 1] : [VACC_EHPSDisable_flg]
    Still -> Normal [order 1] : [!VACC_EHPSDisable_flg]
    Normal -> Error [order 2] : [VACC_EHPSSpdDemTimeout_flg]
    ini -> (junction 29) [order 2]
    (junction 29) -> Error : [(!VACC_SASCalFinish_flg)&&(VPMM_EHPSIniFinish_flg)]
  state Step1
    state Enable
      en:
      VACC_InitEHPSEnDem_flg = TRUE;
      VACC_EHPSSpdCtrlMode_enum  = ENUM_EHPSCTRLMODE_STEP1;
    state Disable
      en:
      VACC_InitEHPSEnDem_flg = FALSE;
      VACC_EHPSSpdCtrlMode_enum  = ENUM_EHPSCTRLMODE_STEP1;
    Enable -> Disable : [VACC_EHPSDisable_flg]
    Disable -> Enable : [!VACC_EHPSDisable_flg]
  state SW
  (default) -> SW
  SW -> Enable [order 2]
  SW -> ini [order 1] : [KACC_EHPSCtrlModeStep2_flg]
  Step2 -> SW : [!KACC_EHPSCtrlModeStep2_flg]
  Step1 -> ini : [KACC_EHPSCtrlModeStep2_flg]
  data: VACC_SASCalFinish_flg input boolean; VPMM_EHPSIniFinish_flg input boolean; VACC_EHPSSpdDemTimeout_flg input boolean; VACC_EHPSDisable_flg input boolean; FALSE parameter; TRUE parameter; VACC_InitEHPSEnDem_flg output boolean; VACC_EHPSSpdCtrlMode_enum output int8; VACC_EBSBrakeRelease_flg input boolean; ENUM_EHPSCTRLMODE_FULLPWR parameter; ENUM_EHPSCTRLMODE_NORMAL parameter; ENUM_EHPSCTRLMODE_ZERO parameter; KACC_EHPSCtrlModeStep2_flg input boolean; ENUM_EHPSCTRLMODE_STEP1 parameter; cnt local single; VINP_EHPSMotorSpdSta_rpm input; KACC_EHPSDisWaitTime_s parameter; KACC_EHPSSpdDiv_rpm parameter; task_time_s input
